simulink library "lib_energy_storage2"  (Simulink 10.1)
settings: Solver=VariableStepAuto  StartTime=0.0  StopTime=10.0  RelTol=1e-3
undefined symbols (not defined in the file or in its folder): air_cp, amb_tmp, cyc_mph, enable_stop, ess_cap_scale, ess_cb, ess_cc, ess_coulombic_eff, ess_init_soc, ess_max_ah_cap, ess_max_p, ess_max_p_soc, ess_max_soc, ess_max_volts, ess_min_soc, ess_min_volts, ess_MMi, ess_MMo, ess_mod_airflow, ess_mod_cp, ess_mod_cpm, ess_mod_init_tmp, ess_module_mass, ess_module_num, ess_on, ess_parallel_mod_num, ess_res_scale_coef, ess_res_scale_fun, ess_set_tmp, ess_soc, ess_th_calc, ess_th_res, ess_th_res_off, ess_th_res_on, ess_tmp, ess_voc, fund_byu, fund_byuop, mc_min_volts, saber_air_temp, Saber_Battery_IO_File, saber_init_soc, saber_init_temp, saber_init_voc, saber_k_cb, saber_k_cc, saber_k_rc, saber_k_re, saber_k_rt, saber_k_soc, t_soc, time_step
undefined symbols (not defined in the file): ess_r_chg, ess_r_dis, ess_rc, ess_re, ess_rt, logFlag
libraries: simulink3 x16, lib_energy_storage x1, $bdroot x1
(part 1 of 8)
Description:
  | energy storage
settings Model: Creator=NREL  LastModifiedBy=sateeshk  ModifiedComment=mzolot -- Mon Apr 29 15:28:23 2002 -- Version 3.0107
settings Model: ModifiedHistory=|
  | mzolot -- Mon Apr 29 15:28:23 2002 -- Version 3.0107
  | 
  | 
  | mzolot -- Mon Apr 29 15:28:23 2002 -- Version 3.0107
  | 
  | 
  | mzolot -- Mon Apr 29 15:09:57 2002 -- Version 3.0106
  | 
  | 
  | mzolot -- Mon Apr 29 14:58:03 2002 -- Version 3.0105
  | 
  | 
  | mzolot -- Mon Apr 29 14:03:19 2002 -- Version 3.0104
  | 
  | 
  | mzolot -- Mon Apr 29 14:02:44 2002 -- Version 3.0103
  | 
  | 
  | mzolot -- Mon Apr 29 14:02:36 2002 -- Version 3.0102
  | 
  | 
  | mzolot -- Mon Apr 29 14:01:30 2002 -- Version 3.0101
  | 
  | 
  | mzolot -- Tue Apr 23 09:34:07 2002 -- Version 3.0100
  | 
  | 
  | mzolot -- Tue Apr 23 09:26:47 2002 -- Version 3.099
  | 
  | 
  | mzolot -- Tue Apr 23 09:26:41 2002 -- Version 3.098
  | 
  | 
  | mzolot -- Fri Apr 19 16:37:41 2002 -- Version 3.097
  | 
  | 
  | mzolot -- Fri Apr 19 11:13:38 2002 -- Version 3.096
  | 
  | 
  | mzolot -- Thu Apr 18 17:16:22 2002 -- Version 3.095
  | 
  | 
  | mokeefe -- Thu Apr 18 08:28:08 2002 -- Version 3.094
  | saving the model:
  | o "without the model browser open"
  | o with only top-level screen visible
  | o with "fit to view" enabled
  | o with "status bar" off and "toolbar" off
  | o with "prompt to update model history with each save" on
  | 
  | vjohnson -- Thu Jan 25 10:35:56 2001 -- Version 3.02
  | 
  | 
  | ssprik -- Wed Nov 01 15:28:33 2000 -- Version 3.01
  | enabled comment dialogue to prompt the person saving the model to add comments.

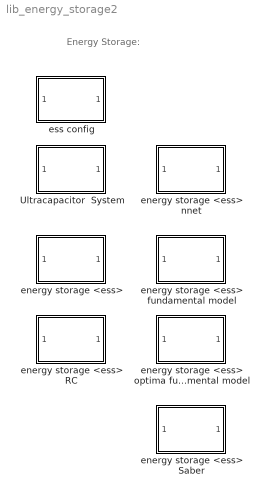
== system lib_energy_storage2 ==
  note: Energy Storage:
  Ultracapacitor  System : Subsystem  mask(Stand-Alone Energy Storage System Mask){generalName='ess', logPick=Log Variable, initFileName={}, modCell={}, imgFileName='bdi_ess.jpg', DEBUG=OFF}
      mask prompts: generalName "General Name of this Component [char]"; logPick "Log Variables to Workspace?"; initFileName "Initialization File(s) [cell array of char]"; modCell "Modification Cell [2 column cell array of param and val]"; imgFileName "Icon image file name [char--evaluated]"
      mask init:
      | % initialization via m-file script
      | advSACompMaskInit;
      mask TypeOptions logPick: Don't Log | Log Variable
      mask TypeOptions DEBUG: ON | OFF
      mask Display: image(imread(imgFileName))
  energy storage <ess> : Subsystem  mask(Stand-Alone Energy Storage System Mask){generalName='ess', logPick=Log Variable, initFileName={}, modCell={}, imgFileName='bdi_ess.jpg', DEBUG=OFF}
      mask prompts: generalName "General Name of this Component [char]"; logPick "Log Variables to Workspace?"; initFileName "Initialization File(s) [cell array of char]"; modCell "Modification Cell [2 column cell array of param and val]"; imgFileName "Icon image file name [char--evaluated]"
      mask init:
      | % initialization via m-file script
      | advSACompMaskInit;
      mask TypeOptions logPick: Don't Log | Log Variable
      mask TypeOptions DEBUG: ON | OFF
      mask Display: image(imread(imgFileName))
  energy storage <ess> RC : Subsystem  mask(Stand-Alone Energy Storage System Mask){generalName='ess', logPick=Log Variable, initFileName={}, modCell={}, imgFileName='bdi_ess.jpg', DEBUG=OFF}
      mask prompts: generalName "General Name of this Component [char]"; logPick "Log Variables to Workspace?"; initFileName "Initialization File(s) [cell array of char]"; modCell "Modification Cell [2 column cell array of param and val]"; imgFileName "Icon image file name [char--evaluated]"
      mask init:
      | % initialization via m-file script
      | advSACompMaskInit;
      mask TypeOptions logPick: Don't Log | Log Variable
      mask TypeOptions DEBUG: ON | OFF
      mask Display: image(imread(imgFileName))
  energy storage <ess> nnet : Subsystem  mask(Stand-Alone Energy Storage System Mask){generalName='ess', logPick=Log Variable, initFileName={}, modCell={}, imgFileName='bdi_ess.jpg', DEBUG=OFF}
      mask prompts: generalName "General Name of this Component [char]"; logPick "Log Variables to Workspace?"; initFileName "Initialization File(s) [cell array of char]"; modCell "Modification Cell [2 column cell array of param and val]"; imgFileName "Icon image file name [char--evaluated]"
      mask init:
      | % initialization via m-file script
      | advSACompMaskInit;
      mask TypeOptions logPick: Don't Log | Log Variable
      mask TypeOptions DEBUG: ON | OFF
      mask Display: image(imread(imgFileName))
  energy storage <ess> Saber : Subsystem  mask(Stand-Alone Energy Storage System Mask){generalName='ess', logPick=Log Variable, initFileName={}, modCell={}, imgFileName='bdi_ess.jpg', DEBUG=OFF}
      mask prompts: generalName "General Name of this Component [char]"; logPick "Log Variables to Workspace?"; initFileName "Initialization File(s) [cell array of char]"; modCell "Modification Cell [2 column cell array of param and val]"; imgFileName "Icon image file name [char--evaluated]"
      mask init:
      | % initialization via m-file script
      | advSACompMaskInit;
      mask TypeOptions logPick: Don't Log | Log Variable
      mask TypeOptions DEBUG: ON | OFF
      mask Display: image(imread(imgFileName))
  energy storage <ess> fundamental model : Subsystem  mask(Stand-Alone Energy Storage System Mask){generalName='ess', logPick=Log Variable, initFileName={}, modCell={}, imgFileName='bdi_ess.jpg', DEBUG=OFF}
      mask prompts: generalName "General Name of this Component [char]"; logPick "Log Variables to Workspace?"; initFileName "Initialization File(s) [cell array of char]"; modCell "Modification Cell [2 column cell array of param and val]"; imgFileName "Icon image file name [char--evaluated]"
      mask init:
      | % initialization via m-file script
      | advSACompMaskInit;
      mask TypeOptions logPick: Don't Log | Log Variable
      mask TypeOptions DEBUG: ON | OFF
      mask Display: image(imread(imgFileName))
  energy storage <ess> optima fundamental model : Subsystem  mask(Stand-Alone Energy Storage System Mask){generalName='ess', logPick=Log Variable, initFileName={}, modCell={}, imgFileName='bdi_ess.jpg', DEBUG=OFF}
      mask prompts: generalName "General Name of this Component [char]"; logPick "Log Variables to Workspace?"; initFileName "Initialization File(s) [cell array of char]"; modCell "Modification Cell [2 column cell array of param and val]"; imgFileName "Icon image file name [char--evaluated]"
      mask init:
      | % initialization via m-file script
      | advSACompMaskInit;
      mask TypeOptions logPick: Don't Log | Log Variable
      mask TypeOptions DEBUG: ON | OFF
      mask Display: image(imread(imgFileName))
  ess config : Subsystem  BlockChoice=energy storage <ess>
      settings: TemplateBlock=self  MemberBlocks="Ultracapacitor  System,energy storage <ess>,energy storage <ess> RC,energy storage <ess> nnet,energy storage <ess> Saber,energy storage <ess> fundamental model,energy storage <ess> optima fundamental model"

== system lib_energy_storage2/Ultracapacitor  System ==
  note: Energy Storage System
  power req'd into bus (W) : Inport
  Block NOTES : Subsystem
      mask Display: disp('Block\nNOTES')
  Ultracapacitor  System : Subsystem
      mask Display: image(imread('bdi_ess.jpg'))
  documentation9 : Subsystem
      settings: OpenFcn=web(['file:\\\' which('energy_storage.htm')]);
      mask Display: image(imread('doc_man.jpg'))
  power available to bus (W) : Outport  InitialOutput=0
  tag scope: essReqOut=global, essSensors=global
  wires:
  power req'd into bus (W)/1 -> Ultracapacitor  System/1(power req'd into bus (W))
  [essControl] -> Ultracapacitor  System/2(control)
  Ultracapacitor  System/1(required out) -> [essReqOut]
  Ultracapacitor  System/2(power available to bus (W)) -> power available to bus (W)/1
  Ultracapacitor  System/3(sensors) -> [essSensors]

== system lib_energy_storage2/energy storage <ess> ==
  note: Energy Storage System
  power req'd into bus (W) : Inport
  Block NOTES : Subsystem
      mask Display: disp('Block\nNOTES')
  documentation9 : Subsystem
      settings: OpenFcn=web(['file:\\\' which('energy_storage.htm')]);
      mask Display: image(imread('doc_man.jpg'))
  energy storage <ess> : Subsystem
      mask Display: image(imread('bdi_ess.jpg'))
  power available to bus (W) : Outport  InitialOutput=0
  tag scope: essReqOut=global, essSensors=global
  wires:
  power req'd into bus (W)/1 -> energy storage <ess>/1(power req'd into bus (W))
  [essControl] -> energy storage <ess>/2(control)
  energy storage <ess>/1(required out) -> [essReqOut]
  energy storage <ess>/2(power available to bus (W)) -> power available to bus (W)/1
  energy storage <ess>/3(sensors) -> [essSensors]

== system lib_energy_storage2/energy storage <ess> RC ==
  note: Energy Storage System
  power req'd into bus (W) : Inport
  Block NOTES : Subsystem
      mask Display: disp('Block\nNOTES')
  documentation9 : Subsystem
      settings: OpenFcn=web(['file:\\\' which('energy_storage.htm')]);
      mask Display: image(imread('doc_man.jpg'))
  energy storage <ess> RC : Subsystem
      mask Display: image(imread('bdi_ess.jpg'))
  power available to bus (W) : Outport  InitialOutput=0
  tag scope: essReqOut=global, essSensors=global
  wires:
  power req'd into bus (W)/1 -> energy storage <ess> RC/1(power req'd into bus (W))
  [essControl] -> energy storage <ess> RC/2(control)
  energy storage <ess> RC/1(required out) -> [essReqOut]
  energy storage <ess> RC/2(power available to bus (W)) -> power available to bus (W)/1
  energy storage <ess> RC/3(sensors) -> [essSensors]

== system lib_energy_storage2/energy storage <ess> nnet ==
  note: Energy Storage System
  power req'd into bus (W) : Inport
  Block NOTES : Subsystem
      mask Display: disp('Block\nNOTES')
  documentation9 : Subsystem
      settings: OpenFcn=web(['file:\\\' which('energy_storage.htm')]);
      mask Display: image(imread('doc_man.jpg'))
  energy storage <ess> nnet : Subsystem
      mask Display: image(imread('bdi_ess.jpg'))
  power available to bus (W) : Outport  InitialOutput=0
  tag scope: essReqOut=global, essSensors=global
  wires:
  power req'd into bus (W)/1 -> energy storage <ess> nnet/1(power req'd into bus (W))
  [essControl] -> energy storage <ess> nnet/2(control)
  energy storage <ess> nnet/1(required out) -> [essReqOut]
  energy storage <ess> nnet/2(power available to bus (W)) -> power available to bus (W)/1
  energy storage <ess> nnet/3(sensors) -> [essSensors]

== system lib_energy_storage2/energy storage <ess> Saber ==
  note: Energy Storage System
  power req'd into bus (W) : Inport
  Block NOTES : Subsystem
      mask Display: disp('Block\nNOTES')
  documentation9 : Subsystem
      settings: OpenFcn=web(['file:\\\' which('energy_storage.htm')]);
      mask Display: image(imread('doc_man.jpg'))
  energy storage <ess> Saber : Subsystem
      mask Display: image(imread('bdi_ess.jpg'))
  power available to bus (W) : Outport  InitialOutput=0
  tag scope: essReqOut=global, essSensors=global
  wires:
  power req'd into bus (W)/1 -> energy storage <ess> Saber/1(power req'd into bus (W))
  [essControl] -> energy storage <ess> Saber/2(control)
  energy storage <ess> Saber/1(required out) -> [essReqOut]
  energy storage <ess> Saber/2(power available to bus (W)) -> power available to bus (W)/1
  energy storage <ess> Saber/3(sensors) -> [essSensors]

== system lib_energy_storage2/energy storage <ess> fundamental model ==
  note: Energy Storage System
  power req'd into bus (W) : Inport
  Block NOTES : Subsystem
      mask Display: disp('Block\nNOTES')
  documentation9 : Subsystem
      settings: OpenFcn=web(['file:\\\' which('energy_storage.htm')]);
      mask Display: image(imread('doc_man.jpg'))
  energy storage <ess> fundamental model : Subsystem
      mask Display: image(imread('bdi_ess.jpg'))
  power available to bus (W) : Outport  InitialOutput=0
  tag scope: essReqOut=global, essSensors=global
  wires:
  power req'd into bus (W)/1 -> energy storage <ess> fundamental model/1(power req'd into bus (W))
  [essControl] -> energy storage <ess> fundamental model/2(control)
  energy storage <ess> fundamental model/1(required out) -> [essReqOut]
  energy storage <ess> fundamental model/2(power available to bus (W)) -> power available to bus (W)/1
  energy storage <ess> fundamental model/3(sensors) -> [essSensors]

== system lib_energy_storage2/energy storage <ess> optima fundamental model ==
  note: Energy Storage System
  power req'd into bus (W) : Inport
  Block NOTES : Subsystem
      mask Display: disp('Block\nNOTES')
  documentation9 : Subsystem
      settings: OpenFcn=web(['file:\\\' which('energy_storage.htm')]);
      mask Display: image(imread('doc_man.jpg'))
  energy storage <ess> optima fundamental model : Subsystem
      mask Display: image(imread('bdi_ess.jpg'))
  power available to bus (W) : Outport  InitialOutput=0
  tag scope: essReqOut=global, essSensors=global
  wires:
  power req'd into bus (W)/1 -> energy storage <ess> optima fundamental model/1(power req'd into bus (W))
  [essControl] -> energy storage <ess> optima fundamental model/2(control)
  energy storage <ess> optima fundamental model/1(required out) -> [essReqOut]
  energy storage <ess> optima fundamental model/2(power available to bus (W)) -> power available to bus (W)/1
  energy storage <ess> optima fundamental model/3(sensors) -> [essSensors]

== system lib_energy_storage2/ess config ==
  power req'd into bus (W) : Inport
  energy storage <ess> : Subsystem  AncestorBlock=lib_energy_storage2/energy storage <ess>  mask(Stand-Alone IC Energy Storage System Mask){generalName='ess', logPick=Log Variable, initFileName={}, modCell={}, imgFileName='bdi_ess.jpg'}
      mask prompts: generalName "General Name of this Component [char]"; logPick "Log Variables to Workspace?"; initFileName "Initialization File(s) [cell array of char]"; modCell "Modification Cell [2 column cell array of param and val]"; imgFileName "Icon image file name [char--evaluated]"
      mask init:
      | % initialization via m-file function
      | DB=0; % debug off
      | logFlag=advSACompMaskInit(generalName,logPick,initFileName,modCell,DB);
      mask TypeOptions logPick: Don't Log | Log Variable
      mask Display: image(imread(imgFileName))
  power available to bus (W) : Outport
  wires:
  power req'd into bus (W)/1 -> energy storage <ess>/1(power req'd into bus (W))
  energy storage <ess>/1(power available to bus (W)) -> power available to bus (W)/1

== system lib_energy_storage2/Ultracapacitor  System/Block NOTES ==
  note: This is a stand-alone version of an energy storage system
      |
      | Several different models are available

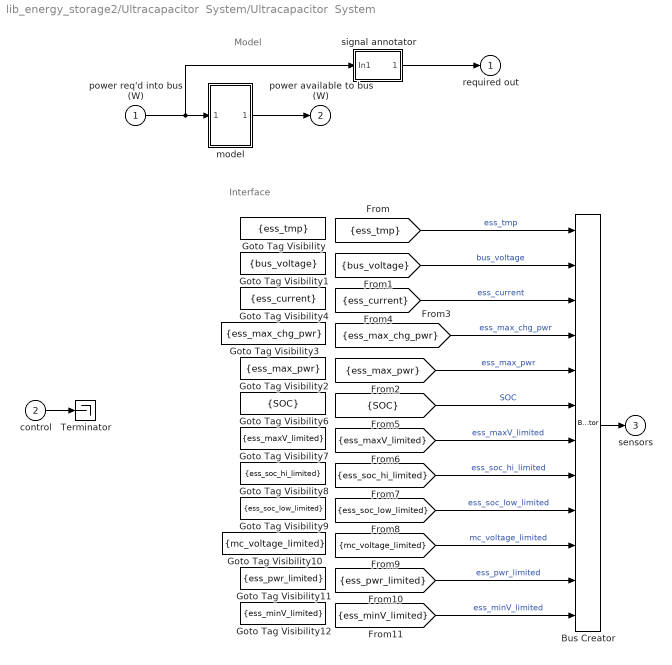
== system lib_energy_storage2/Ultracapacitor  System/Ultracapacitor  System ==
  note: Interface
  note: Model
  power req'd into bus (W) : Inport
  control : Inport  Port=2
  Bus Creator : BusCreator  Inputs=12
  Goto Tag Visibility : GotoTagVisibility  GotoTag=ess_tmp
  Goto Tag Visibility1 : GotoTagVisibility  GotoTag=bus_voltage
  Goto Tag Visibility10 : GotoTagVisibility  GotoTag=mc_voltage_limited
  Goto Tag Visibility11 : GotoTagVisibility  GotoTag=ess_pwr_limited
  Goto Tag Visibility12 : GotoTagVisibility  GotoTag=ess_minV_limited
  Goto Tag Visibility2 : GotoTagVisibility  GotoTag=ess_max_pwr
  Goto Tag Visibility3 : GotoTagVisibility  GotoTag=ess_max_chg_pwr
  Goto Tag Visibility4 : GotoTagVisibility  GotoTag=ess_current
  Goto Tag Visibility6 : GotoTagVisibility  GotoTag=SOC
  Goto Tag Visibility7 : GotoTagVisibility  GotoTag=ess_maxV_limited
  Goto Tag Visibility8 : GotoTagVisibility  GotoTag=ess_soc_hi_limited
  Goto Tag Visibility9 : GotoTagVisibility  GotoTag=ess_soc_low_limited
  Terminator : Terminator
  model : Subsystem
  signal annotator : Subsystem
  required out : Outport  InitialOutput=0
  power available to bus (W) : Outport  Port=2  InitialOutput=0
  sensors : Outport  Port=3  InitialOutput=0
  wires:
  power req'd into bus (W)/1 -> signal annotator/1(In1), model/1(power req'd into bus (W))
  model/1(power available to bus (W)) -> power available to bus (W)/1
  [ess_tmp] -> Bus Creator/1  "ess_tmp"
  control/1 -> Terminator/1
  Bus Creator/1 -> sensors/1
  [bus_voltage] -> Bus Creator/2  "bus_voltage"
  [ess_current] -> Bus Creator/3  "ess_current"
  [ess_max_chg_pwr] -> Bus Creator/4  "ess_max_chg_pwr"
  [ess_max_pwr] -> Bus Creator/5  "ess_max_pwr"
  [SOC] -> Bus Creator/6  "SOC"
  [ess_maxV_limited] -> Bus Creator/7  "ess_maxV_limited"
  [ess_soc_hi_limited] -> Bus Creator/8  "ess_soc_hi_limited"
  [ess_soc_low_limited] -> Bus Creator/9  "ess_soc_low_limited"
  [mc_voltage_limited] -> Bus Creator/10  "mc_voltage_limited"
  [ess_pwr_limited] -> Bus Creator/11  "ess_pwr_limited"
  [ess_minV_limited] -> Bus Creator/12  "ess_minV_limited"
  signal annotator/1(Out1) -> required out/1

== system lib_energy_storage2/Ultracapacitor  System/documentation9 ==

== system lib_energy_storage2/energy storage <ess>/Block NOTES ==
  note: This is a stand-alone version of an energy storage system
      |
      | Several different models are available

== system lib_energy_storage2/energy storage <ess>/documentation9 ==

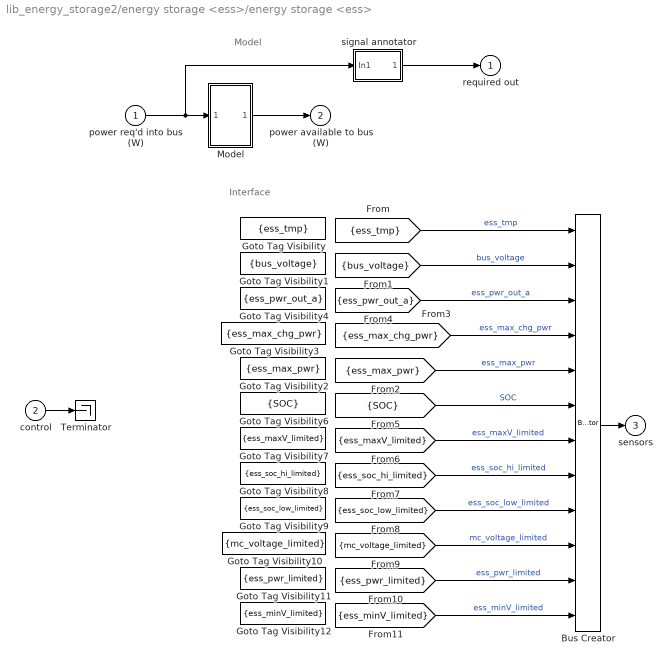
== system lib_energy_storage2/energy storage <ess>/energy storage <ess> ==
  note: Interface
  note: Model
  power req'd into bus (W) : Inport
  control : Inport  Port=2
  Bus Creator : BusCreator  Inputs=12
  Goto Tag Visibility : GotoTagVisibility  GotoTag=ess_tmp
  Goto Tag Visibility1 : GotoTagVisibility  GotoTag=bus_voltage
  Goto Tag Visibility10 : GotoTagVisibility  GotoTag=mc_voltage_limited
  Goto Tag Visibility11 : GotoTagVisibility  GotoTag=ess_pwr_limited
  Goto Tag Visibility12 : GotoTagVisibility  GotoTag=ess_minV_limited
  Goto Tag Visibility2 : GotoTagVisibility  GotoTag=ess_max_pwr
  Goto Tag Visibility3 : GotoTagVisibility  GotoTag=ess_max_chg_pwr
  Goto Tag Visibility4 : GotoTagVisibility  GotoTag=ess_pwr_out_a
  Goto Tag Visibility6 : GotoTagVisibility  GotoTag=SOC
  Goto Tag Visibility7 : GotoTagVisibility  GotoTag=ess_maxV_limited
  Goto Tag Visibility8 : GotoTagVisibility  GotoTag=ess_soc_hi_limited
  Goto Tag Visibility9 : GotoTagVisibility  GotoTag=ess_soc_low_limited
  Model : Subsystem
  Terminator : Terminator
  signal annotator : Subsystem
  required out : Outport  InitialOutput=0
  power available to bus (W) : Outport  Port=2  InitialOutput=0
  sensors : Outport  Port=3  InitialOutput=0
  wires:
  power req'd into bus (W)/1 -> Model/1(power req'd into bus (W)), signal annotator/1(In1)
  Model/1(power available to bus (W)) -> power available to bus (W)/1
  [ess_tmp] -> Bus Creator/1  "ess_tmp"
  control/1 -> Terminator/1
  Bus Creator/1 -> sensors/1
  [bus_voltage] -> Bus Creator/2  "bus_voltage"
  [ess_pwr_out_a] -> Bus Creator/3  "ess_pwr_out_a"
  [ess_max_chg_pwr] -> Bus Creator/4  "ess_max_chg_pwr"
  [ess_max_pwr] -> Bus Creator/5  "ess_max_pwr"
  [SOC] -> Bus Creator/6  "SOC"
  [ess_maxV_limited] -> Bus Creator/7  "ess_maxV_limited"
  [ess_soc_hi_limited] -> Bus Creator/8  "ess_soc_hi_limited"
  [ess_soc_low_limited] -> Bus Creator/9  "ess_soc_low_limited"
  [mc_voltage_limited] -> Bus Creator/10  "mc_voltage_limited"
  [ess_pwr_limited] -> Bus Creator/11  "ess_pwr_limited"
  [ess_minV_limited] -> Bus Creator/12  "ess_minV_limited"
  signal annotator/1(Out1) -> required out/1

== system lib_energy_storage2/energy storage <ess> RC/Block NOTES ==
  note: This is a stand-alone version of an energy storage system
      |
      | Several different models are available

== system lib_energy_storage2/energy storage <ess> RC/documentation9 ==

== system lib_energy_storage2/energy storage <ess> RC/energy storage <ess> RC ==
  note: Interface
  note: Model
  power req'd into bus (W) : Inport
  control : Inport  Port=2
  Bus Creator : BusCreator  Inputs=5
  Goto Tag Visibility : GotoTagVisibility  GotoTag=ess_tmp
  Goto Tag Visibility1 : GotoTagVisibility  GotoTag=bus_voltage
  Goto Tag Visibility2 : GotoTagVisibility  GotoTag=ess_max_pwr
  Goto Tag Visibility3 : GotoTagVisibility  GotoTag=ess_max_chg_pwr
  Goto Tag Visibility6 : GotoTagVisibility  GotoTag=SOC
  Terminator : Terminator
  model : Subsystem
  signal annotator : Subsystem
  required out : Outport  InitialOutput=0
  power available to bus (W) : Outport  Port=2  InitialOutput=0
  sensors : Outport  Port=3  InitialOutput=0
  wires:
  power req'd into bus (W)/1 -> signal annotator/1(In1), model/1(power req'd into bus (W))
  model/1(power available to bus (W)) -> power available to bus (W)/1
  control/1 -> Terminator/1
  Bus Creator/1 -> sensors/1
  signal annotator/1(Out1) -> required out/1
  [ess_tmp] -> Bus Creator/1  "ess_tmp"
  [bus_voltage] -> Bus Creator/2  "bus_voltage"
  [ess_max_chg_pwr] -> Bus Creator/3  "ess_max_chg_pwr"
  [ess_max_pwr] -> Bus Creator/4  "ess_max_pwr"
  [SOC] -> Bus Creator/5  "SOC"

== system lib_energy_storage2/energy storage <ess> nnet/Block NOTES ==
  note: This is a stand-alone version of an energy storage system
      |
      | Several different models are available

== system lib_energy_storage2/energy storage <ess> nnet/documentation9 ==

== system lib_energy_storage2/energy storage <ess> nnet/energy storage <ess> nnet ==
  note: Interface
  note: Model
  power req'd into bus (W) : Inport
  control : Inport  Port=2
  Bus Creator : BusCreator  Inputs=8
  Goto Tag Visibility1 : GotoTagVisibility  GotoTag=bus_voltage
  Goto Tag Visibility10 : GotoTagVisibility  GotoTag=mc_voltage_limited
  Goto Tag Visibility11 : GotoTagVisibility  GotoTag=ess_pwr_limited
  Goto Tag Visibility12 : GotoTagVisibility  GotoTag=ess_minV_limited
  Goto Tag Visibility2 : GotoTagVisibility  GotoTag=ess_max_pwr
  Goto Tag Visibility6 : GotoTagVisibility  GotoTag=SOC
  Goto Tag Visibility7 : GotoTagVisibility  GotoTag=ess_maxV_limited
  Goto Tag Visibility8 : GotoTagVisibility  GotoTag=ess_soc_limited
  Terminator : Terminator
  model : Subsystem
  signal annotator : Subsystem
  required out : Outport  InitialOutput=0
  power available to bus (W) : Outport  Port=2  InitialOutput=0
  sensors : Outport  Port=3  InitialOutput=0
  wires:
  power req'd into bus (W)/1 -> signal annotator/1(In1), model/1(power req'd into bus (W))
  model/1(power available to bus (W)) -> power available to bus (W)/1
  control/1 -> Terminator/1
  Bus Creator/1 -> sensors/1
  signal annotator/1(Out1) -> required out/1
  [bus_voltage] -> Bus Creator/1  "bus_voltage"
  [ess_max_pwr] -> Bus Creator/2  "ess_max_pwr"
  [SOC] -> Bus Creator/3  "SOC"
  [ess_maxV_limited] -> Bus Creator/4  "ess_maxV_limited"
  [ess_soc_limited] -> Bus Creator/5  "ess_soc_limited"
  [mc_voltage_limited] -> Bus Creator/6  "mc_voltage_limited"
  [ess_pwr_limited] -> Bus Creator/7  "ess_pwr_limited"
  [ess_minV_limited] -> Bus Creator/8  "ess_minV_limited"

== system lib_energy_storage2/energy storage <ess> Saber/Block NOTES ==
  note: This is a stand-alone version of an energy storage system
      |
      | Several different models are available

== system lib_energy_storage2/energy storage <ess> Saber/documentation9 ==

== system lib_energy_storage2/energy storage <ess> Saber/energy storage <ess> Saber ==
  note: Interface
  note: Model
  power req'd into bus (W) : Inport
  control : Inport  Port=2
  Bus Creator : BusCreator  Inputs=3
  Goto Tag Visibility1 : GotoTagVisibility  GotoTag=bus_voltage
  Goto Tag Visibility2 : GotoTagVisibility  GotoTag=ess_max_pwr
  Goto Tag Visibility6 : GotoTagVisibility  GotoTag=SOC
  Terminator : Terminator
  model : Subsystem
  signal annotator : Subsystem
  required out : Outport  InitialOutput=0
  power available to bus (W) : Outport  Port=2  InitialOutput=0
  sensors : Outport  Port=3  InitialOutput=0
  wires:
  power req'd into bus (W)/1 -> signal annotator/1(In1), model/1(power req'd into bus (W))
  model/1(power available to bus (W)) -> power available to bus (W)/1
  control/1 -> Terminator/1
  Bus Creator/1 -> sensors/1
  signal annotator/1(Out1) -> required out/1
  [bus_voltage] -> Bus Creator/1  "bus_voltage"
  [ess_max_pwr] -> Bus Creator/2  "ess_max_pwr"
  [SOC] -> Bus Creator/3  "SOC"

== system lib_energy_storage2/energy storage <ess> fundamental model/Block NOTES ==
  note: This is a stand-alone version of an energy storage system
      |
      | Several different models are available

== system lib_energy_storage2/energy storage <ess> fundamental model/documentation9 ==

== system lib_energy_storage2/energy storage <ess> fundamental model/energy storage <ess> fundamental model ==
  note: Interface
  note: Model
  power req'd into bus (W) : Inport
  control : Inport  Port=2
  Bus Creator : BusCreator  Inputs=3
  Goto Tag Visibility1 : GotoTagVisibility  GotoTag=bus_voltage
  Goto Tag Visibility2 : GotoTagVisibility  GotoTag=ess_max_pwr
  Goto Tag Visibility6 : GotoTagVisibility  GotoTag=SOC
  Terminator : Terminator
  model : Subsystem
  signal annotator : Subsystem
  required out : Outport  InitialOutput=0
  power available to bus (W) : Outport  Port=2  InitialOutput=0
  sensors : Outport  Port=3  InitialOutput=0
  wires:
  power req'd into bus (W)/1 -> signal annotator/1(In1), model/1(power req'd into bus (W))
  model/1(power available to bus (W)) -> power available to bus (W)/1
  control/1 -> Terminator/1
  Bus Creator/1 -> sensors/1
  signal annotator/1(Out1) -> required out/1
  [bus_voltage] -> Bus Creator/1  "bus_voltage"
  [ess_max_pwr] -> Bus Creator/2  "ess_max_pwr"
  [SOC] -> Bus Creator/3  "SOC"

== system lib_energy_storage2/energy storage <ess> optima fundamental model/Block NOTES ==
  note: This is a stand-alone version of an energy storage system
      |
      | Several different models are available

== system lib_energy_storage2/energy storage <ess> optima fundamental model/documentation9 ==

== system lib_energy_storage2/energy storage <ess> optima fundamental model/energy storage <ess> optima fundamental model ==
  note: Interface
  note: Model
  power req'd into bus (W) : Inport
  control : Inport  Port=2
  Bus Creator : BusCreator  Inputs=3
  Goto Tag Visibility1 : GotoTagVisibility  GotoTag=bus_voltage
  Goto Tag Visibility2 : GotoTagVisibility  GotoTag=ess_max_pwr
  Goto Tag Visibility6 : GotoTagVisibility  GotoTag=SOC
  Terminator : Terminator
  model : Subsystem
  signal annotator : Subsystem
  required out : Outport  InitialOutput=0
  power available to bus (W) : Outport  Port=2  InitialOutput=0
  sensors : Outport  Port=3  InitialOutput=0
  wires:
  power req'd into bus (W)/1 -> signal annotator/1(In1), model/1(power req'd into bus (W))
  model/1(power available to bus (W)) -> power available to bus (W)/1
  control/1 -> Terminator/1
  Bus Creator/1 -> sensors/1
  [ess_max_pwr] -> Bus Creator/2  "ess_max_pwr"
  [SOC] -> Bus Creator/3  "SOC"
  signal annotator/1(Out1) -> required out/1
  [bus_voltage] -> Bus Creator/1  "bus_voltage"

== system lib_energy_storage2/ess config/energy storage <ess> ==
  note: Energy Storage System
  power req'd into bus (W) : Inport
  Block NOTES : Subsystem
      mask Display: disp('Block\nNOTES')
  Ultracapacitor  System : $bdroot/Ess Choices/Ultracapacitor  System
  documentation9 : Subsystem
      settings: OpenFcn=web(['file:\\\' which('energy_storage.htm')]);
      mask Display: image(imread('doc_man.jpg'))
  power available to bus (W) : Outport  InitialOutput=0
  tag scope: essReqOut=global, essSensors=global
  wires:
  Ultracapacitor  System/3 -> [essSensors]
  Ultracapacitor  System/2 -> power available to bus (W)/1
  Ultracapacitor  System/1 -> [essReqOut]
  [essControl] -> Ultracapacitor  System/2
  power req'd into bus (W)/1 -> Ultracapacitor  System/1
